simulink model "controlador_ppi"  (R2021a)
settings: Solver=ode15s  StartTime=0.0  StopTime=2*pi  RelTol=1e-3
model workspace (MAT data in the model file):
  wn = 1.57079632679
values from neighbouring files (symbols this model uses):
  M_bar = zeros(7, 7)    [kinova_gen3.m]
libraries: roblocks x1
settings Model: Creator=Lucas  LastModifiedBy=Lucas

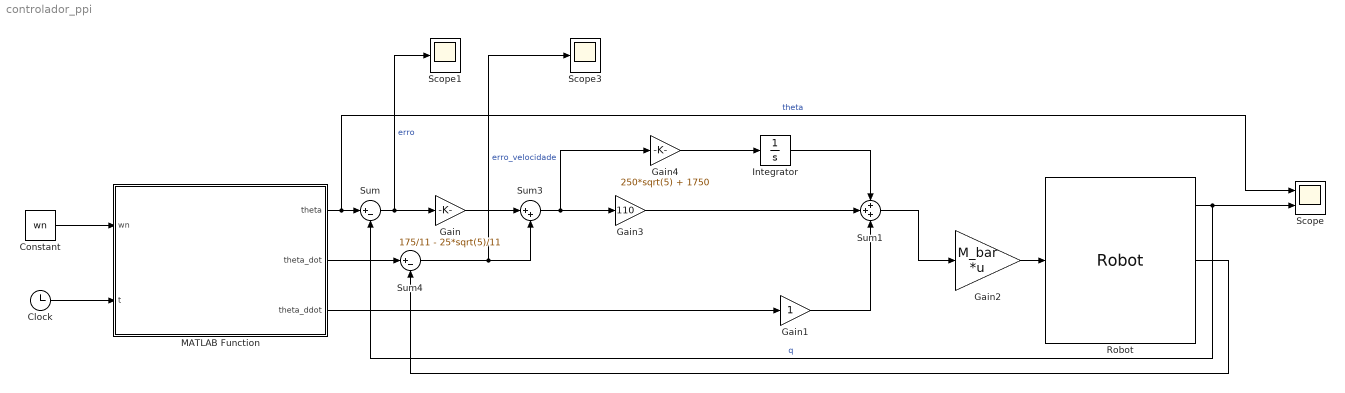
== system controlador_ppi ==
  Clock : Clock
  Constant : Constant  Value=wn
  Gain : Gain  Gain=175/11 - 25*sqrt(5)/11
  Gain1 : Gain
  Gain2 : Gain  Gain=M_bar  Multiplication=Matrix(K*u)
  Gain3 : Gain  Gain=110
  Gain4 : Gain  Gain=250*sqrt(5) + 1750
  Integrator : Integrator
  MATLAB Function : MATLAB Function  TreatAsAtomicUnit=on
  Robot : roblocks/Arm/Robot  robot=kinova  q0=deg2rad([0, 15, 180, -130, 0, 55, 90])
  Scope : Scope  NumInputPorts=2
  Scope1 : Scope
  Scope3 : Scope
  Sum : Sum  Inputs=|+-
  Sum1 : Sum  Inputs=+++
  Sum3 : Sum  Inputs=|++
  Sum4 : Sum  Inputs=|+-
  wires:
  Constant/1 -> MATLAB Function/1(wn)
  Clock/1 -> MATLAB Function/2(t)
  MATLAB Function/1(theta) -> Sum/1, Scope/1  "theta"
  Robot/1 -> Scope/2, Sum/2  "q"
  Robot/2 -> Sum4/2
  Sum/1 -> Gain/1, Scope1/1  "erro"
  Gain2/1 -> Robot/1
  Sum1/1 -> Gain2/1
  MATLAB Function/2(theta_dot) -> Sum4/1
  Sum4/1 -> Scope3/1, Sum3/2  "erro_velocidade"
  Gain/1 -> Sum3/1
  Sum3/1 -> Gain3/1, Gain4/1
  MATLAB Function/3(theta_ddot) -> Gain1/1
  Gain1/1 -> Sum1/3
  Gain3/1 -> Sum1/2
  Gain4/1 -> Integrator/1
  Integrator/1 -> Sum1/1

== matlab function controlador_ppi/MATLAB Function ==
  data: wn input; theta output; t input; theta_dot output; theta_ddot output
function [theta, theta_dot, theta_ddot] = trajetoria_desejada(wn, t)
    % Função para calcular a trajetória desejada e suas derivadas
    
    % Trajetórias desejadas (em radianos)
    theta = [
        0.5236 * cos(wn * t);                              % θ1d
        0.2618 + 0.2618 * cos(wn * t);                     % θ2d (1)
        pi * ones(size(t));                                % θ2d (2)
        -2.2689 + 0.2618 * cos(1.2 * wn * t);              % θ2d (3)
        zeros(size(t));                                    % θ2d (4)
        0.9599 + 0.2618 * cos(1.3 * wn * t);               % θ2d (5)
        pi/2 * ones(size(t));                              % θ2d (6)
    ];
    
    % Primeira derivada das trajetórias
    theta_dot = [
        -0.5236 * wn * sin(wn * t);                        % θ1d_dot
        -0.2618 * wn * sin(wn * t);                        % θ2d_dot (1)
        zeros(size(t));                                    % θ2d_dot (2)
        -0.2618 * 1.2 * wn * sin(1.2 * wn * t);            % θ2d_dot (3)
        zeros(size(t));                                    % θ2d_dot (4)
        -0.2618 * 1.3 * wn * sin(1.3 * wn * t);            % θ2d_dot (5)
        zeros(size(t));                                    % θ2d_dot (6)
    ];
    
    % Segunda derivada das trajetórias
    theta_ddot = [
        -0.5236 * wn^2 * cos(wn * t);                      % θ1d_ddot
        -0.2618 * wn^2 * cos(wn * t);                      % θ2d_ddot (1)
        zeros(size(t));                                    % θ2d_ddot (2)
        -0.2618 * (1.2 * wn)^2 * cos(1.2 * wn * t);        % θ2d_ddot (3)
        zeros(size(t));                                    % θ2d_ddot (4)
        -0.2618 * (1.3 * wn)^2 * cos(1.3 * wn * t);        % θ2d_ddot (5)
        zeros(size(t));                                    % θ2d_ddot (6)
    ];
end
